simulink model "E2_Simulink"  (R2023a)
settings: Solver=VariableStepAuto  StartTime=0.0  StopTime=0.2  RelTol=1e-3
values from neighbouring files (symbols this model uses):
  b = 0.0012    [E2_Parametros.m]
  j = 0.001    [E2_Parametros.m]
  ke = 0.01    [E2_Parametros.m]
  kt = 0.01    [E2_Parametros.m]
  l = 0.023    [E2_Parametros.m]
  r = 2    [E2_Parametros.m]
  vi = 1    [E2_Parametros.m]
settings Model: Creator=mluser  LastModifiedBy=mluser

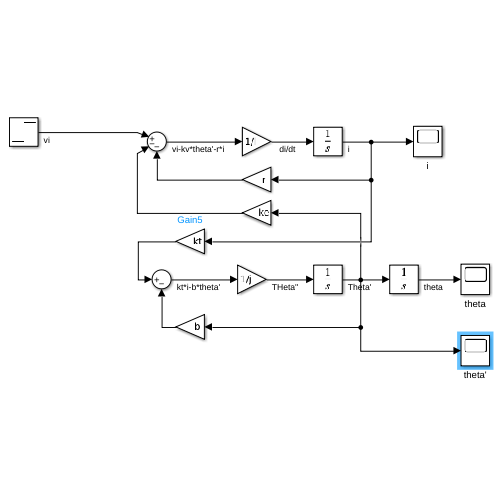
[thumbnail: Simulink's stored preview of the top-level diagram]
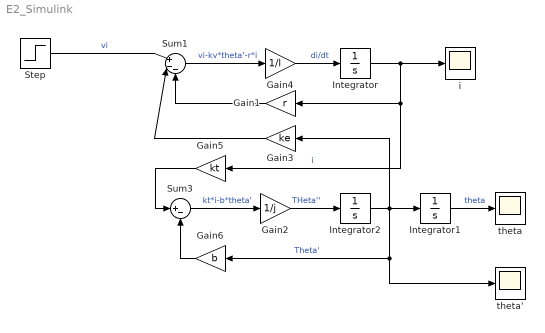
== system E2_Simulink ==
  Gain1 : Gain  Gain=r
  Gain2 : Gain  Gain=1/j
  Gain3 : Gain  Gain=ke
  Gain4 : Gain  Gain=1/l
  Gain5 : Gain  Gain=kt
  Gain6 : Gain  Gain=b
  Integrator : Integrator
  Integrator1 : Integrator
  Integrator2 : Integrator
  Step : Step  Time=0  After=vi  SampleTime=0
  Sum1 : Sum  Inputs=|+--
  Sum3 : Sum  Inputs=|+-
  i : Scope
  theta : Scope
  theta' : Scope
  wires:
  Step/1 -> Sum1/1  "vi"
  Gain4/1 -> Integrator/1  "di/dt"
  Sum1/1 -> Gain4/1  "vi-kv*theta'-r*i"
  Integrator/1 -> Gain1/1, Gain5/1, i/1  "i"
  Integrator1/1 -> theta/1  "theta"
  Integrator2/1 -> theta'/1, Gain6/1, Gain3/1, Integrator1/1  "Theta'"
  Gain2/1 -> Integrator2/1  "THeta''"
  Sum3/1 -> Gain2/1  "kt*i-b*theta'"
  Gain1/1 -> Sum1/3
  Gain3/1 -> Sum1/2
  Gain5/1 -> Sum3/1
  Gain6/1 -> Sum3/2
